simulink model "Labo2_parte2si"  (R2025b)
settings: Solver=FixedStepAuto  StartTime=0.0  StopTime=10  RelTol=1e-3  EnableMultiTasking=on
undefined symbols (not defined in the file or in its folder): ss8, ss9
libraries: arduinolib x3, arduinosensorlib x1
settings Model: ExtModeTrigDuration=2  Creator=ALIENWARE-GAMER  LastModifiedBy=Froilán Pardo
settings SolverCC: AutoInsertRateTranBlk=on
settings OptimizationCC: BlockReduction=off  BooleanDataType=off  EnhancedBackFolding=on  PassReuseOutputArgsAs=Individual arguments  ZeroExternalMemoryAtStartup=off  ZeroInternalMemoryAtStartup=off  MaxStackSize=64  OptimizeBlockOrder=speed  DifferentSizesBufferReuse=on  OptimizationCustomize=off  EfficientTunableParamExpr=on
settings DebuggingCC: SaveWithParameterizedLinksMsg=none  UnderspecifiedInitializationDetection=Classic  MergeDetectMultiDrivingBlocksExec=none  SignalResolutionControl=TryResolveAllWithWarning  ParameterTunabilityLossMsg=error
settings HardwareCC: ProdBitPerInt=16.0  ProdBitPerPointer=16.0  ProdBitPerSizeT=16.0  ProdBitPerPtrDiffT=16.0  ProdLargestAtomicFloat=None  ProdWordSize=8.0  ProdHWDeviceType=Atmel->AVR  TargetBitPerInt=16.0  TargetBitPerPointer=16.0  TargetBitPerSizeT=16.0  TargetBitPerPtrDiffT=16.0  TargetIntDivRoundTo=Zero  TargetEndianess=LittleEndian  TargetWordSize=8.0  TargetHWDeviceType=Atmel->AVR
settings ModelReferenceCC: PropagateSignalLabelsOutOfModel=off
settings SFSimCC: MATLABDynamicMemAlloc=off
settings RTWCC: SystemTargetFile=ert.tlc  HardwareBoard=Arduino Uno  TemplateMakefile=ert_default_tmf  Toolchain=Arduino AVR  BuildConfiguration=Faster Runs  Description=Embedded Coder
settings CodeAppCC: ForceParamTrailComments=on  IgnoreCustomStorageClasses=off  OperatorAnnotations=on  SimulinkDataObjDesc=on  SFDataObjDesc=on  InsertBlockDesc=on
settings ERTTargetCC: ExtModeTransport=3.0  ExtModeStaticAlloc=on  ExtModeAutomaticAllocSize=off  ExtModeStaticAllocSize=250.0  ExtModeMexFile=ext_xcp  ExtModeIntrfLevel=Level2 - Open  InlinedParameterPlacement=Hierarchical  SupportContinuousTime=on  SupportVariableSizeSignals=on

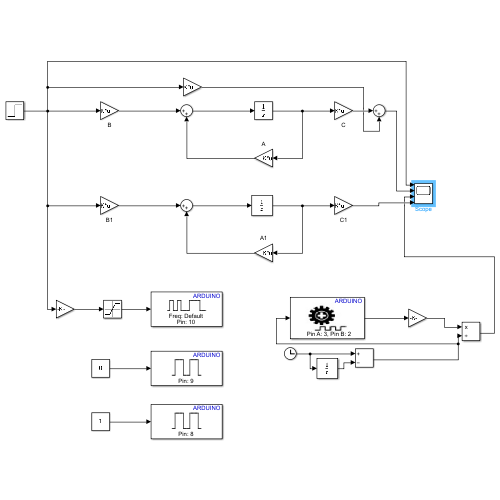
[thumbnail: Simulink's stored preview of the top-level diagram]
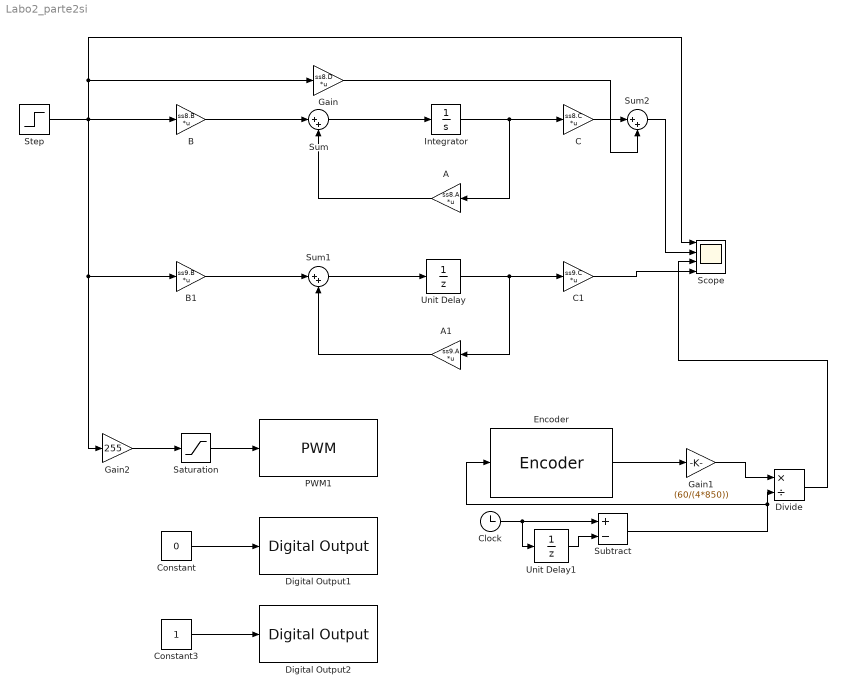
== system Labo2_parte2si ==
  A : Gain  Gain=ss8.A  Multiplication=Matrix(K*u)
  A1 : Gain  Gain=ss9.A  Multiplication=Matrix(K*u)
  B : Gain  Gain=ss8.B  Multiplication=Matrix(K*u)
  B1 : Gain  Gain=ss9.B  Multiplication=Matrix(K*u)
  C : Gain  Gain=ss8.C  Multiplication=Matrix(K*u)
  C1 : Gain  Gain=ss9.C  Multiplication=Matrix(K*u)
  Clock : Clock
  Constant : Constant  Value=0
  Constant3 : Constant
  Digital Output1 : arduinolib/Digital Output  pinNumber=9  Direction=output  blockPlatform=arduino
  Digital Output2 : arduinolib/Digital Output  pinNumber=8  Direction=output  blockPlatform=arduino
  Divide : Product  Inputs=*/
  Encoder : arduinosensorlib/Encoder  InputA=3  InputB=2  Mode=Reset by external signal  SampleTime=-1
  Gain : Gain  Gain=ss8.D  Multiplication=Matrix(K*u)
  Gain1 : Gain  Gain=(60/(4*850))
  Gain2 : Gain  Gain=255
  Integrator : Integrator  InitialCondition=[0 0]
  PWM1 : arduinolib/PWM  pinNumber=10  frequencyType=Default  desiredFrequency=490.2  achievableFrequency=490.2
  Saturation : Saturate  UpperLimit=255  LowerLimit=0
  Scope : Scope  NumInputPorts=4
      settings: ActiveDisplayYMinimum=-301.04264831542969  ActiveDisplayYMaximum=586.44560241699219
  Step : Step  SampleTime=0
  Subtract : Sum  Inputs=+-
  Sum : Sum  Inputs=|++
  Sum1 : Sum  Inputs=|++
  Sum2 : Sum  Inputs=|++
  Unit Delay : UnitDelay  SampleTime=-1  HasFrameUpgradeWarning=on
  Unit Delay1 : UnitDelay  SampleTime=-1  HasFrameUpgradeWarning=on
  wires:
  B/1 -> Sum/1
  Sum/1 -> Integrator/1
  Integrator/1 -> A/1, C/1
  A/1 -> Sum/2
  Unit Delay/1 -> A1/1, C1/1
  B1/1 -> Sum1/1
  A1/1 -> Sum1/2
  C1/1 -> Scope/4
  Sum1/1 -> Unit Delay/1
  C/1 -> Sum2/1
  Gain/1 -> Sum2/2
  Sum2/1 -> Scope/2
  Step/1 -> Scope/1, Gain/1, Gain2/1, B1/1, B/1
  Clock/1 -> Subtract/1, Unit Delay1/1
  Gain1/1 -> Divide/1
  Unit Delay1/1 -> Subtract/2
  Encoder/1 -> Gain1/1
  Subtract/1 -> Divide/2, Encoder/1
  Divide/1 -> Scope/3
  Constant/1 -> Digital Output1/1
  Constant3/1 -> Digital Output2/1
  Gain2/1 -> Saturation/1
  Saturation/1 -> PWM1/1
